simulink model "Part4_2_5_new"  (R2021a)
settings: Solver=VariableStepAuto  StartTime=0.0  StopTime=100  RelTol=1e-3
settings Model: Creator=theod  LastModifiedBy=theod

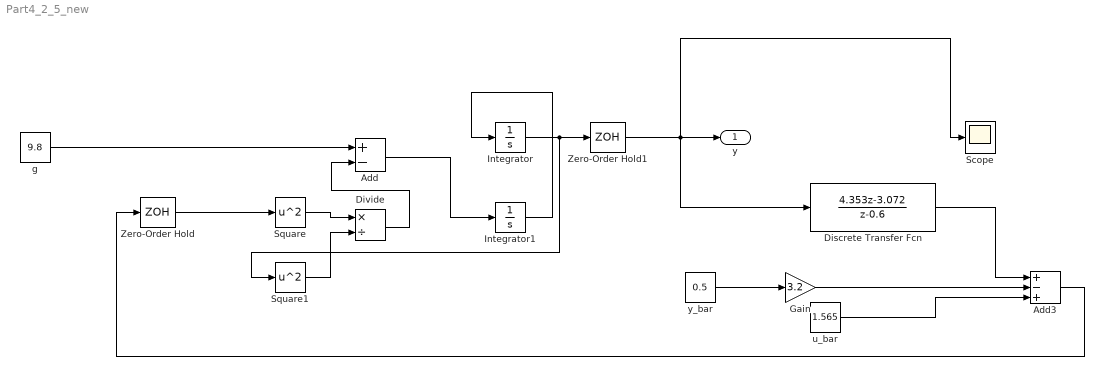
== system Part4_2_5_new ==
  Add : Sum  Inputs=+-
  Add3 : Sum  Inputs=+-+
  Discrete Transfer Fcn : DiscreteTransferFcn  Numerator=[4.353 -3.072]  Denominator=[1 -0.6]
  Divide : Product  Inputs=*/
  Gain : Gain  Gain=3.2
  Integrator : Integrator  InitialCondition=11
  Integrator1 : Integrator  InitialCondition=2
  Scope : Scope
  Square : Math  Operator=square  SaturateOnIntegerOverflow=on
  Square1 : Math  Operator=square  SaturateOnIntegerOverflow=on
  Zero-Order Hold : ZeroOrderHold  SampleTime=-1
  Zero-Order Hold1 : ZeroOrderHold  SampleTime=0.05
  g : Constant  Value=9.8
  u_bar : Constant  Value=1.565
  y_bar : Constant  Value=0.5
  y : Outport
  wires:
  Integrator1/1 -> Integrator/1
  Integrator/1 -> Square1/1, Zero-Order Hold1/1
  Square/1 -> Divide/1
  Square1/1 -> Divide/2
  Divide/1 -> Add/2
  g/1 -> Add/1
  Add/1 -> Integrator1/1
  u_bar/1 -> Add3/3
  Zero-Order Hold/1 -> Square/1
  Add3/1 -> Zero-Order Hold/1
  Zero-Order Hold1/1 -> Scope/1, Discrete Transfer Fcn/1, y/1
  Discrete Transfer Fcn/1 -> Add3/1
  y_bar/1 -> Gain/1
  Gain/1 -> Add3/2
